simulink model "TestLogOptoforce2017"  (R2017b)
settings: Solver=FixedStepDiscrete  StartTime=0.0  StopTime=inf  FixedStep=0.01  RelTol=1e-3  EnableMultiTasking=on
undefined symbols (not defined in the file or in its folder): serial
libraries: robotlib x3, etargetslib x2, instrumentlib x2
settings Model: Creator=mine  LastModifiedBy=BCI-USER
settings DataIOCC: LimitDataPoints=on  SaveFormat=Array
settings OptimizationCC: LifeSpan=inf
settings DebuggingCC: UnderspecifiedInitializationDetection=Classic  MergeDetectMultiDrivingBlocksExec=none  SolverPrmCheckMsg=warning  StateNameClashWarn=warning  SFUnexpectedBacktrackingDiag=warning  SFNoUnconditionalDefaultTransitionDiag=warning  SFExecutionAtInitializationDiag=none
settings HardwareCC: ProdBitPerPointer=32  ProdBitPerSizeT=32  ProdBitPerPtrDiffT=32  ProdLargestAtomicFloat=None  ProdIntDivRoundTo=Undefined  ProdEndianess=Unspecified  ProdWordSize=32  ProdHWDeviceType=32-bit Generic
settings ModelReferenceCC: PropagateSignalLabelsOutOfModel=off
settings CodeAppCC: StateflowObjectComments=on
settings GRTTargetCC: TargetLangStandard=C89/C90 (ANSI)  GeneratePreprocessorConditionals=Disable all
settings ConfigComp: CovMetricSettings=dw  CovHtmlReporting=on  CovSaveCumulativeToWorkspaceVar=on  CovSaveSingleToWorkspaceVar=on  CovExternalEMLEnable=off

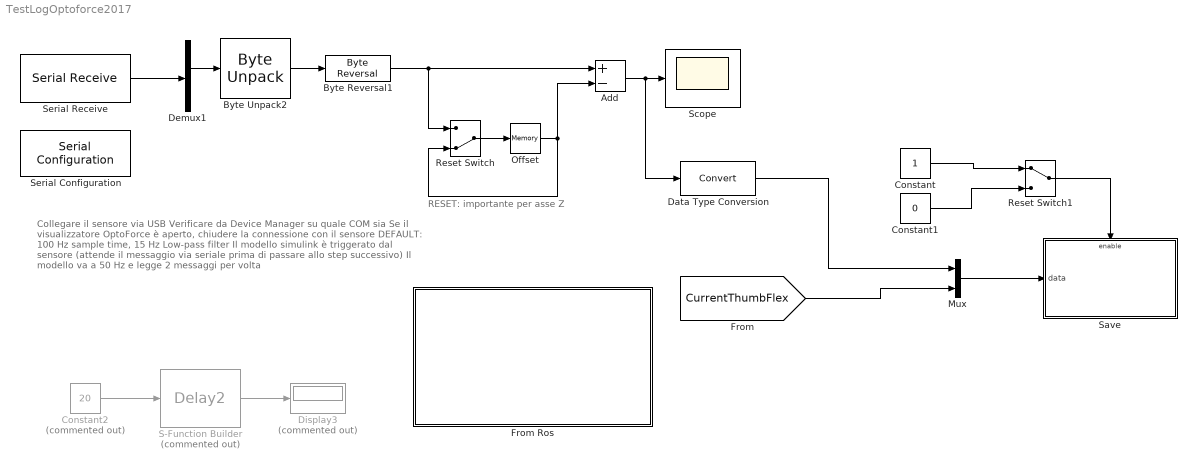
== system TestLogOptoforce2017 ==
  note: RESET: importante per asse Z
  note: Collegare il sensore via USB
      | Verificare da Device Manager su quale COM sia
      | Se il visualizzatore OptoForce è aperto, chiudere la connessione con il sensore
      |
      | DEFAULT: 100 Hz sample time, 15 Hz Low-pass filter
      |
      | Il modello simulink è triggerato dal sensore
      | (attende il messaggio via seriale prima di passare allo step successivo)
      | Il modello va a 50 Hz e legge 2 messaggi per volta
  Add : Sum  Inputs=+-
  Byte Reversal1 : etargetslib/Byte Reversal  numInp=1
  Byte Unpack2 : etargetslib/Byte Unpack  dimensions={3}  datatypes={'int16'}  byteAlign=1
  Constant : Constant
  Constant1 : Constant  Value=0
  Constant2 : Constant  Commented=on  Value=20  OutDataTypeStr=uint32  SampleTime=-1
  Data Type Conversion : DataTypeConversion
  Demux1 : Demux  Outputs="[3 6 20  29]"
  Display3 : Display  Commented=on
  From Ros : Subsystem
  Mux : Mux  Inputs=2
  Offset : Memory  InitialCondition=[0 0 0]
  Reset Switch : ManualSwitch  CurrentSetting=0
  Reset Switch1 : ManualSwitch
  S-Function Builder : S-Function  Commented=on  InitFcn=try, set_param(gcb,'FunctionName','Delay2'), end  FunctionName=Delay2  SFunctionModules=Delay2_wrapper  SFunctionDeploymentMode=off  EnableBusSupport=off  mask(S-Function Builder){}
      mask help: Simulink:masks:SFunctionBuilder_MD
      mask init:
      | val = [[.9  0.75 0.75 1 1 .9 .9 1]',[1 1 0.75 0.75 .9 .9 1 .9]'];try , sys = get_param(gcb,'SfunBuilderFcnName');if isempty(sys), sys = get_param(gcb,'FunctionName'); end,catch, sys = get_param(gcb,'FunctionName'); end
      settings: CopyFcn=set_param(gcbh,'LinkStatus','none')  PreSaveFcn=try, set_param(gcb,'FunctionName','Delay2'), end  OpenFcn=sfunctionwizard(gcbh)
      mask Display: plot(val(:,1),val(:,2)),disp(sys), port_label('input',1,'u0'), port_label('output',1,'y0')
  Save : Subsystem
  Scope : Scope
  Serial Configuration : instrumentlib/Serial Configuration  Priority=-200000  ComPortMenu=COM2  ComPort=COM2  ObjConstructor=serial('COM2');  BaudRate=115200  DataBits=8  Parity=none  StopBits=1  FlowControl=none  Timeout=5  ByteOrder=LittleEndian
  Serial Receive : instrumentlib/Serial Receive  ComPortMenu=COM2  ComPort=COM2  ObjConstructor=serial('COM2');  Terminator=<none>  DataSize="[58   1]"  DataType=uint8  EnableBlockingMode=on  ActionDataUnavailable=Output last received value  CustomValue=0  SampleTime=-1
  wires:
  Constant2/1 -> S-Function Builder/1
  S-Function Builder/1 -> Display3/1
  Serial Receive/1 -> Demux1/1
  Byte Unpack2/1 -> Byte Reversal1/1
  Demux1/2 -> Byte Unpack2/1
  Byte Reversal1/1 -> Reset Switch/1, Add/1
  Add/1 -> Data Type Conversion/1, Scope/1
  Reset Switch/1 -> Offset/1
  Offset/1 -> Reset Switch/2, Add/2
  [CurrentThumbFlex] -> Mux/2
  Data Type Conversion/1 -> Mux/1
  Mux/1 -> Save/1(data)
  Constant/1 -> Reset Switch1/1
  Constant1/1 -> Reset Switch1/2
  Reset Switch1/1 -> Save/Enable

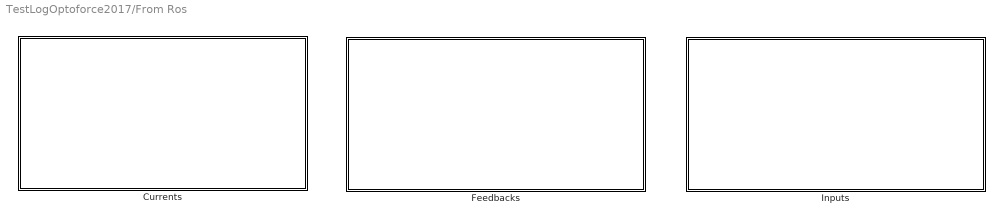
== system TestLogOptoforce2017/From Ros ==
  Currents : Subsystem
  Feedbacks : Subsystem
  Inputs : Subsystem

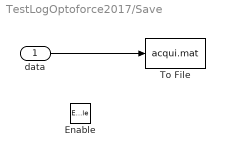
== system TestLogOptoforce2017/Save ==
  data : Inport
  Enable : EnablePort
  To File : ToFile  Filename=acqui.mat
  wires:
  data/1 -> To File/1

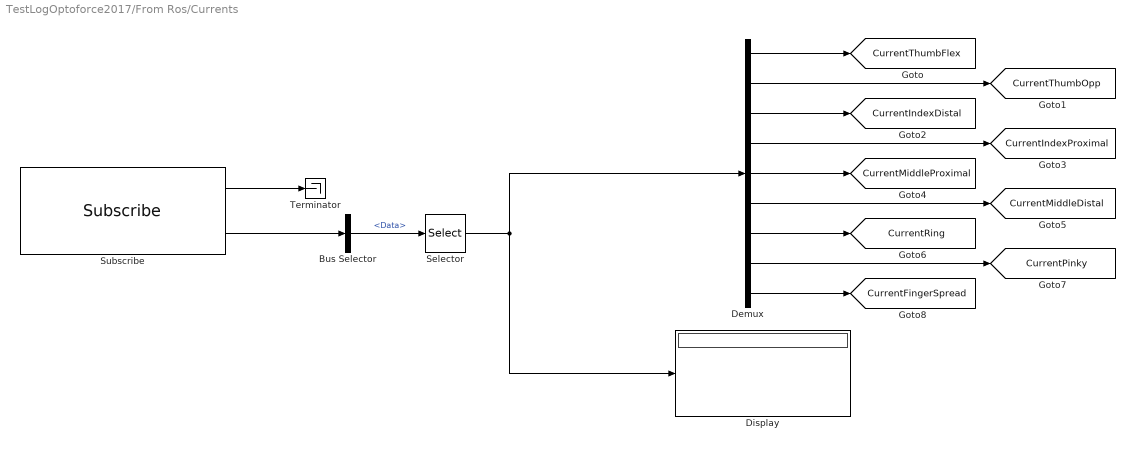
== system TestLogOptoforce2017/From Ros/Currents ==
  Bus Selector : BusSelector  OutputSignals=Data
  Demux : Demux  Outputs=9
  Display : Display
  Selector : Selector  IndexOptions=Index vector (dialog)  Indices=[1 2 3 4 5 6 7 8 9]  OutputSizes=1
  Subscribe : robotlib/Subscribe  SourceLibraryInfo=This block requires Robotics System Toolbox  topicSource=Select from ROS network  topic=/svh_controller/channel_currents  messageType=std_msgs/Float64MultiArray  sampleTime=0.01  messageQueueLength=1
      settings: SourceProductBaseCode=RO
  Terminator : Terminator
  tag scope: CurrentFingerSpread=global, CurrentIndexDistal=global, CurrentIndexProximal=global, CurrentMiddleDistal=global, CurrentMiddleProximal=global, CurrentPinky=global, CurrentRing=global, CurrentThumbFlex=global, CurrentThumbOpp=global
  wires:
  Subscribe/2 -> Bus Selector/1
  Selector/1 -> Demux/1, Display/1
  Bus Selector/1 -> Selector/1  "<Data>"
  Demux/1 -> [CurrentThumbFlex]
  Demux/4 -> [CurrentIndexProximal]
  Demux/5 -> [CurrentMiddleProximal]
  Demux/7 -> [CurrentRing]
  Subscribe/1 -> Terminator/1
  Demux/2 -> [CurrentThumbOpp]
  Demux/3 -> [CurrentIndexDistal]
  Demux/6 -> [CurrentMiddleDistal]
  Demux/8 -> [CurrentPinky]
  Demux/9 -> [CurrentFingerSpread]

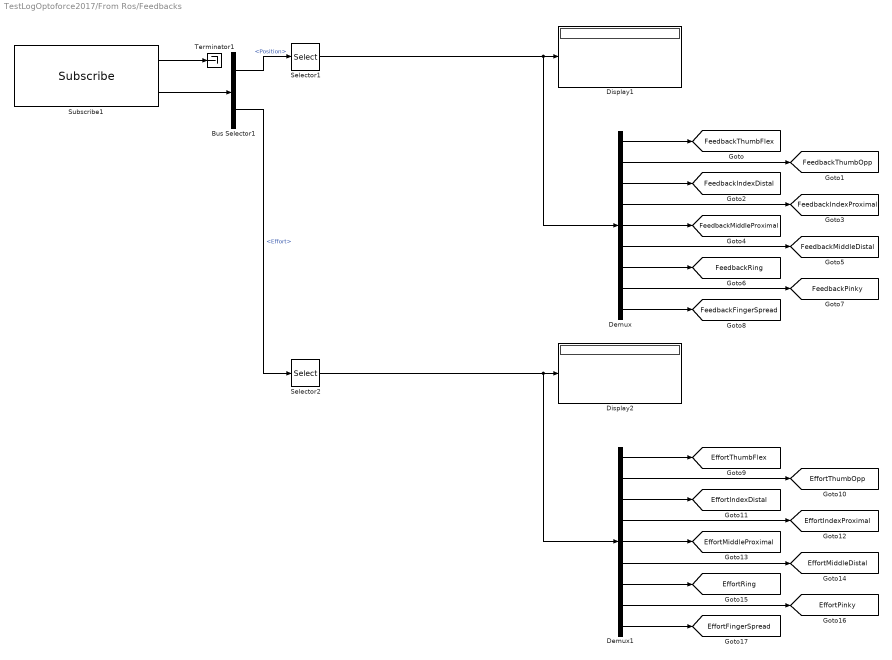
== system TestLogOptoforce2017/From Ros/Feedbacks ==
  Bus Selector1 : BusSelector  OutputSignals=Position,Effort
  Demux : Demux  Outputs=9
  Demux1 : Demux  Outputs=9
  Display1 : Display
  Display2 : Display
  Selector1 : Selector  IndexOptions=Index vector (dialog)  Indices=[1 2 3 4 5 6 7 8 9]  OutputSizes=1
  Selector2 : Selector  IndexOptions=Index vector (dialog)  Indices=[1 2 3 4 5 6 7 8 9]  OutputSizes=1
  Subscribe1 : robotlib/Subscribe  SourceLibraryInfo=This block requires Robotics System Toolbox  topicSource=Select from ROS network  topic=/svh_controller/channel_feedback  messageType=sensor_msgs/JointState  sampleTime=0.01  messageQueueLength=1
      settings: SourceProductBaseCode=RO
  Terminator1 : Terminator
  tag scope: EffortFingerSpread=global, EffortIndexDistal=global, EffortIndexProximal=global, EffortMiddleDistal=global, EffortMiddleProximal=global, EffortPinky=global, EffortRing=global, EffortThumbFlex=global, EffortThumbOpp=global, FeedbackFingerSpread=global, FeedbackIndexDistal=global, FeedbackIndexProximal=global, FeedbackMiddleDistal=global, FeedbackMiddleProximal=global, FeedbackPinky=global, FeedbackRing=global, FeedbackThumbFlex=global, FeedbackThumbOpp=global
  wires:
  Bus Selector1/1 -> Selector1/1  "<Position>"
  Bus Selector1/2 -> Selector2/1  "<Effort>"
  Subscribe1/1 -> Terminator1/1
  Subscribe1/2 -> Bus Selector1/1
  Demux/3 -> [FeedbackIndexDistal]
  Selector1/1 -> Demux/1, Display1/1
  Demux/2 -> [FeedbackThumbOpp]
  Demux/7 -> [FeedbackRing]
  Demux/1 -> [FeedbackThumbFlex]
  Demux/6 -> [FeedbackMiddleDistal]
  Demux/5 -> [FeedbackMiddleProximal]
  Demux/8 -> [FeedbackPinky]
  Demux/9 -> [FeedbackFingerSpread]
  Demux/4 -> [FeedbackIndexProximal]
  Demux1/2 -> [EffortThumbOpp]
  Demux1/5 -> [EffortMiddleProximal]
  Demux1/1 -> [EffortThumbFlex]
  Demux1/6 -> [EffortMiddleDistal]
  Demux1/9 -> [EffortFingerSpread]
  Selector2/1 -> Demux1/1, Display2/1
  Demux1/4 -> [EffortIndexProximal]
  Demux1/7 -> [EffortRing]
  Demux1/8 -> [EffortPinky]
  Demux1/3 -> [EffortIndexDistal]

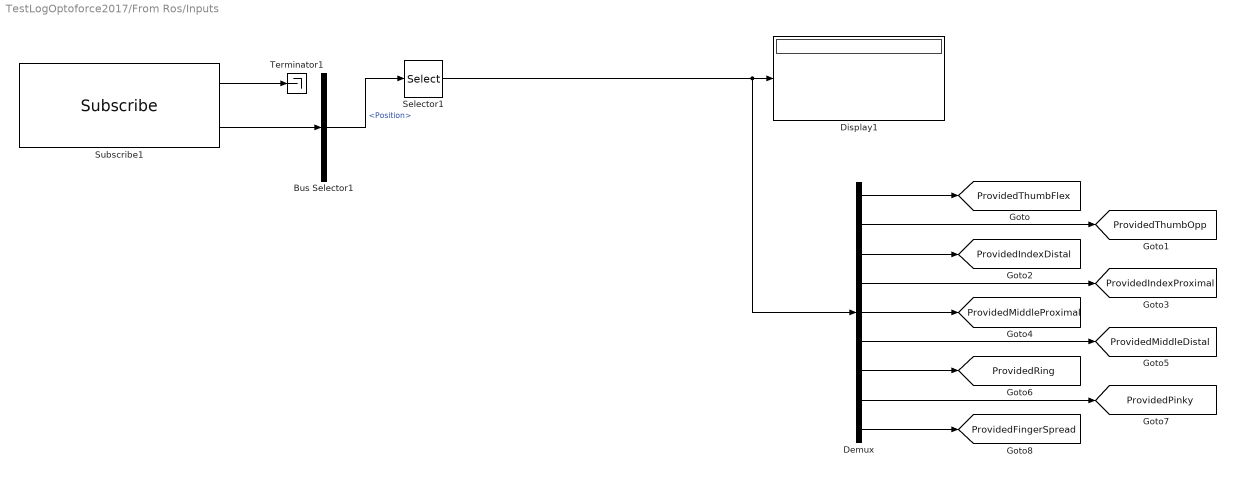
== system TestLogOptoforce2017/From Ros/Inputs ==
  Bus Selector1 : BusSelector  OutputSignals=Position
  Demux : Demux  Outputs=9
  Display1 : Display
  Selector1 : Selector  IndexOptions=Index vector (dialog)  Indices=[1 20 12 8 11 7 6 5 17]  OutputSizes=1
  Subscribe1 : robotlib/Subscribe  SourceLibraryInfo=This block requires Robotics System Toolbox  topicSource=Select from ROS network  topic=/svh_controller/channel_targets  messageType=sensor_msgs/JointState  sampleTime=0.01  messageQueueLength=1
      settings: SourceProductBaseCode=RO
  Terminator1 : Terminator
  tag scope: ProvidedFingerSpread=global, ProvidedIndexDistal=global, ProvidedIndexProximal=global, ProvidedMiddleDistal=global, ProvidedMiddleProximal=global, ProvidedPinky=global, ProvidedRing=global, ProvidedThumbFlex=global, ProvidedThumbOpp=global
  wires:
  Bus Selector1/1 -> Selector1/1  "<Position>"
  Subscribe1/1 -> Terminator1/1
  Subscribe1/2 -> Bus Selector1/1
  Demux/3 -> [ProvidedIndexDistal]
  Selector1/1 -> Demux/1, Display1/1
  Demux/2 -> [ProvidedThumbOpp]
  Demux/7 -> [ProvidedRing]
  Demux/1 -> [ProvidedThumbFlex]
  Demux/6 -> [ProvidedMiddleDistal]
  Demux/5 -> [ProvidedMiddleProximal]
  Demux/8 -> [ProvidedPinky]
  Demux/9 -> [ProvidedFingerSpread]
  Demux/4 -> [ProvidedIndexProximal]
